simulink library "planarTether_ul"  (R2018b)
settings: Solver=VariableStepAuto  StartTime=0.0  StopTime=10.0  RelTol=1e-3
settings Model: Creator=Ayaz  LastModifiedBy=Ayaz

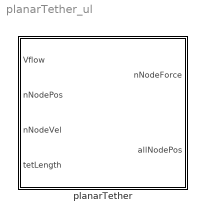
== system planarTether_ul ==
  planarTether : Subsystem  mask{rhoF=1, gravAcc=9.81, numNode=3, tetDia=0.001, tetDensity=1000, tetCD=0.5, tetYoungs=4e9, tetZeta=0.05, mT=100, gndNodePos=[0;0]}
      mask prompts: rhoF "Fluid density"; gravAcc "Gravitational acceleration"; numNode "Number of nodes"; tetDia "Tether diameter"; tetDensity "Tether density"; tetCD "Tether CD"; tetYoungs "Tether Young's modulus"; tetZeta "Tether damping ratio"; mT "Mass of body"; gndNodePos "Ground node position vector"
      mask init:
      | if numNode < 3
      |     numNode = 3;
      | end
      mask DialogControl ParameterGroupVar Prompt: Environment
      mask DialogControl Container3 Prompt: Tether
      mask DialogControl Container4 Prompt: Node locations

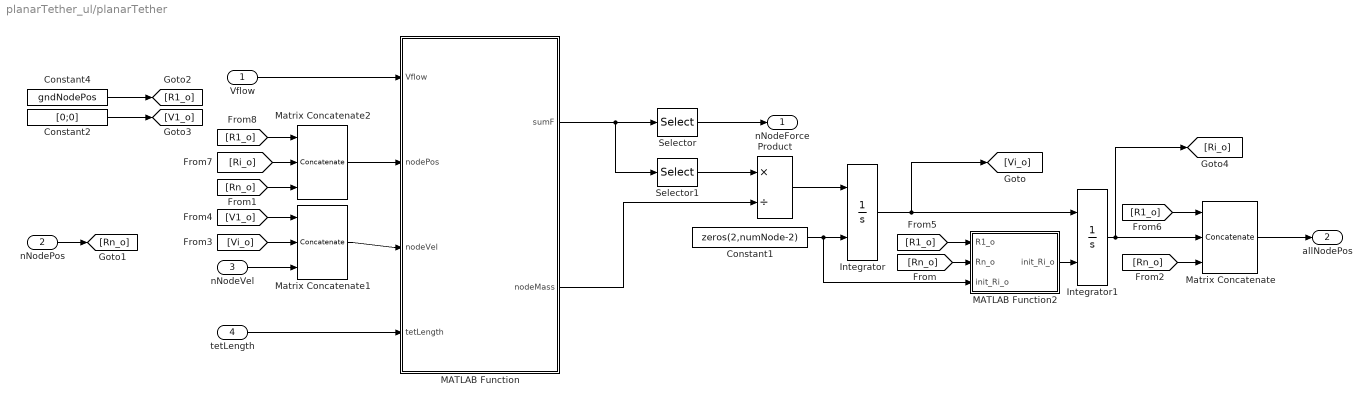
== system planarTether_ul/planarTether ==
  Vflow : Inport  PortDimensions=[2,1]
  nNodePos : Inport  Port=2  PortDimensions=[2,1]
  nNodeVel : Inport  Port=3  PortDimensions=[2,1]
  tetLength : Inport  Port=4  PortDimensions=[1,1]
  Constant1 : Constant  Value=zeros(2,numNode-2)  VectorParams1D=off
  Constant2 : Constant  Value=[0;0]  VectorParams1D=off
  Constant4 : Constant  Value=gndNodePos  VectorParams1D=off
  Integrator : Integrator  InitialConditionSource=external
  Integrator1 : Integrator  InitialConditionSource=external
  MATLAB Function : MATLAB Function  TreatAsAtomicUnit=on
  MATLAB Function2 : MATLAB Function  TreatAsAtomicUnit=on
  Matrix Concatenate : Concatenate  NumInputs=3  Mode=Multidimensional array  ConcatenateDimension=2
  Matrix Concatenate1 : Concatenate  NumInputs=3  Mode=Multidimensional array  ConcatenateDimension=2
  Matrix Concatenate2 : Concatenate  NumInputs=3  Mode=Multidimensional array  ConcatenateDimension=2
  Product : Product  Inputs=*/
  Selector : Selector  NumberOfDimensions=2  InputPortWidth=3  IndexOptions=Select all,Index vector (dialog)  Indices=[1 3],numNode  OutputSizes=1,1
  Selector1 : Selector  NumberOfDimensions=2  InputPortWidth=3  IndexOptions=Select all,Index vector (dialog)  Indices=[1 3],2:numNode-1  OutputSizes=1,1
  nNodeForce : Outport  PortDimensions=[2;1]
  allNodePos : Outport  Port=2  PortDimensions=[2,numNode]
  wires:
  nNodePos/1 -> [Rn_o]
  nNodeVel/1 -> Matrix Concatenate1/3
  tetLength/1 -> MATLAB Function/4(tetLength)
  Vflow/1 -> MATLAB Function/1(Vflow)
  MATLAB Function/1(sumF) -> Selector/1, Selector1/1
  Selector/1 -> nNodeForce/1
  Selector1/1 -> Product/1
  MATLAB Function/2(nodeMass) -> Product/2
  Product/1 -> Integrator/1
  [R1_o] -> MATLAB Function2/1(R1_o)
  MATLAB Function2/1(init_Ri_o) -> Integrator1/2
  [Rn_o] -> MATLAB Function2/2(Rn_o)
  Constant1/1 -> MATLAB Function2/3("init_Ri_o "), Integrator/2
  Integrator/1 -> [Vi_o], Integrator1/1
  Integrator1/1 -> [Ri_o], Matrix Concatenate/2
  [Rn_o] -> Matrix Concatenate/3
  [R1_o] -> Matrix Concatenate/1
  Matrix Concatenate/1 -> allNodePos/1
  Constant4/1 -> [R1_o]
  [V1_o] -> Matrix Concatenate1/1
  [Vi_o] -> Matrix Concatenate1/2
  Matrix Concatenate1/1 -> MATLAB Function/3(nodeVel)
  [Ri_o] -> Matrix Concatenate2/2
  [R1_o] -> Matrix Concatenate2/1
  [Rn_o] -> Matrix Concatenate2/3
  Matrix Concatenate2/1 -> MATLAB Function/2(nodePos)
  Constant2/1 -> [V1_o]

== matlab function planarTether_ul/planarTether/MATLAB Function2 ==
  data: R1_o input; init_Ri_o output; Rn_o input; init_Ri_o input; numNode parameter
function init_Ri_o = fcn(R1_o,Rn_o,init_Ri_o,numNode)

temp= [linspace(R1_o(1),Rn_o(1),numNode);
    linspace(R1_o(2),Rn_o(2),numNode)];

temp(:,1) = [];
temp(:,end) = [];

for ii = 1:numNode-2
    init_Ri_o(:,ii) = temp(:,ii);
end

end

== matlab function planarTether_ul/planarTether/MATLAB Function ==
  data: Vflow input; sumF output size=[2,numNode]; nodePos input size=[2,numNode]; nodeVel input size=[2,numNode]; tetLength input size=[1,1]; nodeMass output size=[1,1]; tetDia parameter; tetDensity parameter; tetYoungs parameter; tetZeta parameter; mT parameter; rhoF parameter; gravAcc parameter; tetCD parameter
function [sumF,nodeMass] = fcn(Vflow,nodePos,nodeVel,tetLength, tetDia, tetDensity,tetYoungs, tetZeta, mT, rhoF, gravAcc, tetCD)
%UNTITLED Summary of this function goes here
%   Detailed explanation goes here

% [sumF,nodeMass] = calcTetForce(Vflow,nodePos,nodeVel,tetLength,numNode,...
%     tetDia,tetDensity,tetCD,tetYoungs,tetZeta,mT,rhoF,gravAcc);

[sumF,nodeMass] = nodeForce(Vflow,nodePos,nodeVel,...
    tetLength,mT,tetZeta,tetDia,tetYoungs,tetCD,rhoF,tetDensity,gravAcc);

end
